simulink model "drone_propre"  (Simulink 6.1)
settings: Solver=ode45  StartTime=0.0  StopTime=10.0  RelTol=1e-3
undefined symbols (not defined in the file): Mecanique
libraries: mblibv1 x15, powerlib x2, electricdrivelib x1
settings Model: LastModifiedBy=Vincent
settings DebuggingCC: SolverPrmCheckMsg=warning

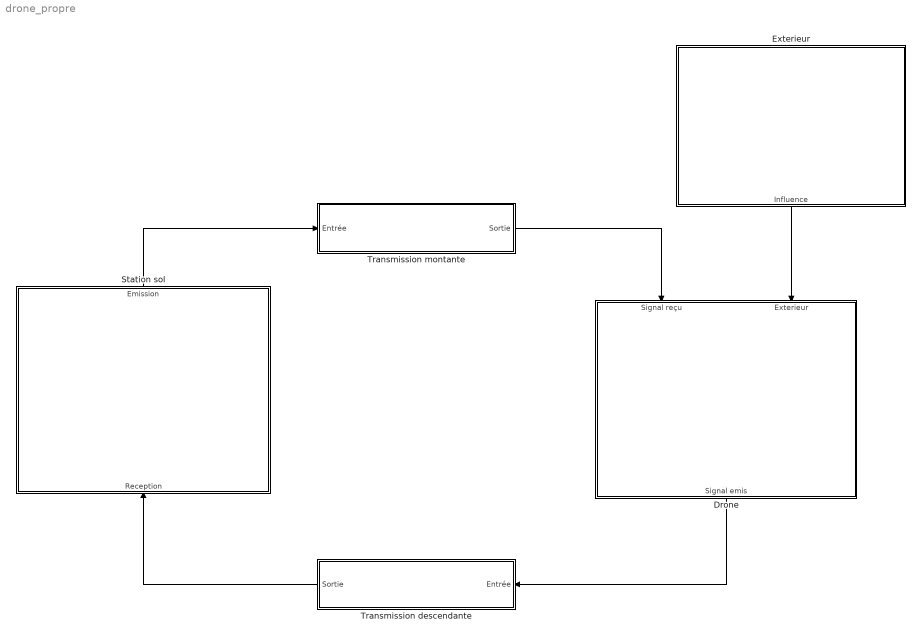
== system drone_propre ==
  Drone : Subsystem  Orientation=down
      mask Display: image(imread('C:\Projets\CMD\Simulations\Propre\images\drone.jpg'))
  Exterieur : Subsystem  Orientation=down
      mask Display: image(imread('C:\Projets\CMD\Simulations\Propre\images\ciel.jpg'))
  Station sol : Subsystem  Orientation=up
      mask Display: image(imread('C:\Projets\CMD\Simulations\Propre\images\stationsol.jpg'))
  Transmission descendante : Subsystem  Orientation=left
      mask Display: image(imread('C:\Projets\CMD\Simulations\Propre\images\ondes2.jpg'))
  Transmission montante : Subsystem
      mask Display: image(imread('C:\Projets\CMD\Simulations\Propre\images\ondes1.jpg'))
  wires:
  Transmission descendante/1(Sortie) -> Station sol/1(Reception)
  Station sol/1(Emission) -> Transmission montante/1(Entrée)
  Transmission montante/1(Sortie) -> Drone/1(Signal reçu)
  Drone/1(Signal emis) -> Transmission descendante/1(Entrée)
  Exterieur/1(Influence) -> Drone/2(Exterieur)

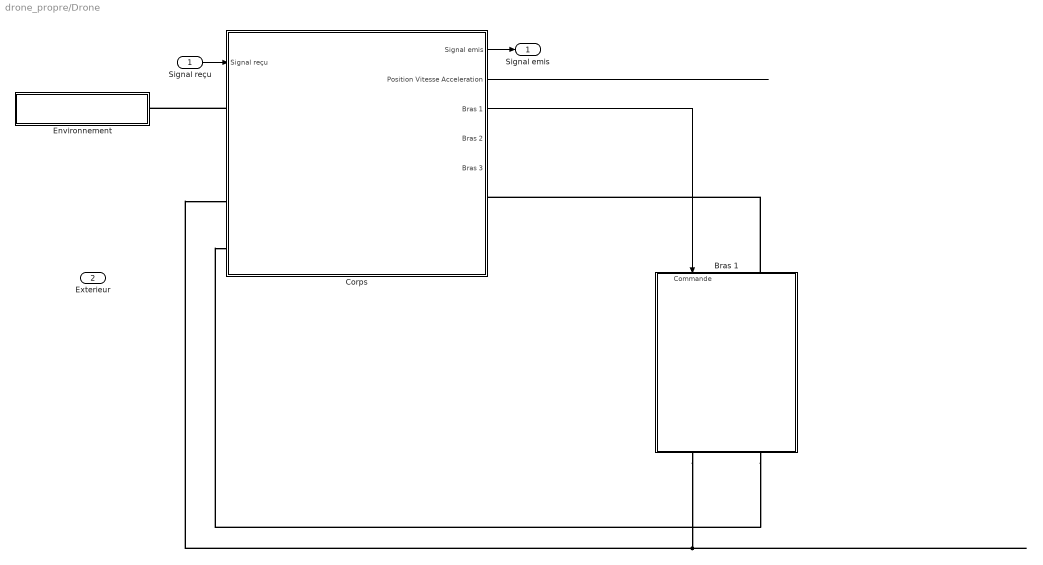
== system drone_propre/Drone ==
  Signal reçu : Inport  Port=1  LatchInput=off
  Exterieur : Inport  Port=2  LatchInput=off
  Bras 1 : Subsystem  Orientation=down
  Corps : Subsystem
  Environnement : Subsystem  Orientation=left
  Signal emis : Outport
  wires:
  Signal reçu/1 -> Corps/1(Signal reçu)
  Corps/1(Signal emis) -> Signal emis/1
  Corps/3(Bras 1) -> Bras 1/1(Commande)
  Corps/2(Position Vitesse Acceleration) -> ?
  connections:
  Corps/LConn1 -- Environnement/LConn1
  Corps/LConn3 -- Bras 1/RConn1
  Bras 1/RConn2 -- Corps/LConn4
  Bras 1/LConn1 -- Corps/RConn1

== system drone_propre/Exterieur ==
  Influence : Outport

== system drone_propre/Station sol ==
  Reception : Inport  Port=1  LatchInput=off
  Emission : Outport
  wires:
  Reception/1 -> Emission/1

== system drone_propre/Transmission descendante ==
  Entrée : Inport  Port=1  LatchInput=off
  Délai de transmission : TransportDelay  DelayTime=1E-4
  Sortie : Outport
  wires:
  Entrée/1 -> Délai de transmission/1
  Délai de transmission/1 -> Sortie/1

== system drone_propre/Transmission montante ==
  Entrée : Inport  Port=1  LatchInput=off
  Délai de transmission : TransportDelay  DelayTime=1E-4
  Sortie : Outport
  wires:
  Entrée/1 -> Délai de transmission/1
  Délai de transmission/1 -> Sortie/1

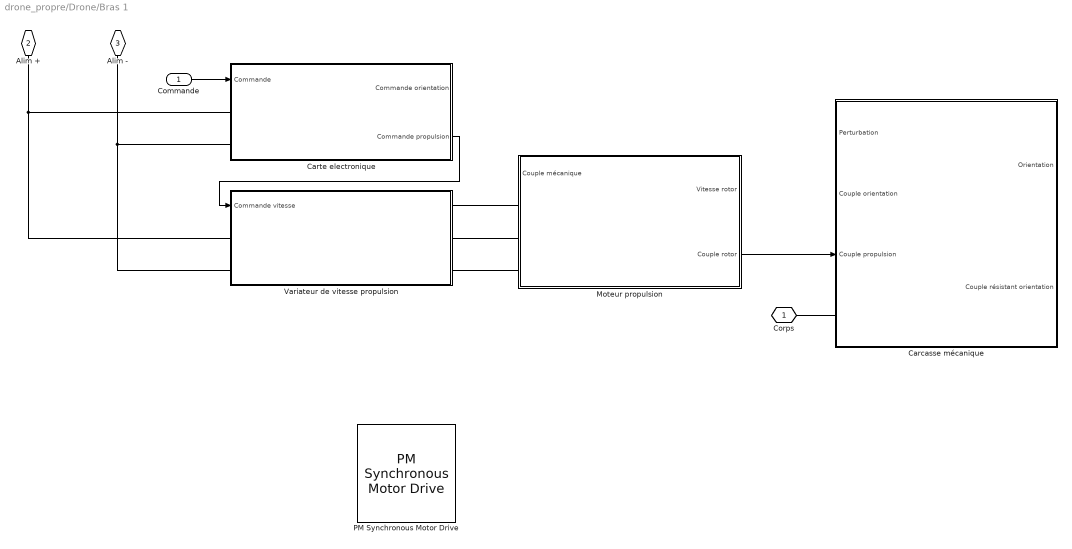
== system drone_propre/Drone/Bras 1 ==
  Commande : Inport  Port=1  LatchInput=off
  Carcasse mécanique : Subsystem
  Carte electronique : Subsystem
  Moteur propulsion : Subsystem
  PM Synchronous Motor Drive : electricdrivelib/AC drives/PM Synchronous Motor Drive
  Variateur de vitesse propulsion : Subsystem
  Corps : PMIOPort  Tag=PMCPort  Port=1  Side=Left
  Alim + : PMIOPort  Tag=PMCPort  Orientation=down  Port=2  Side=Right
  Alim - : PMIOPort  Tag=PMCPort  Orientation=down  Port=3  Side=Right
  wires:
  Moteur propulsion/2(Couple rotor) -> Carcasse mécanique/3(Couple propulsion)
  Commande/1 -> Carte electronique/1(Commande)
  Carte electronique/2(Commande propulsion) -> Variateur de vitesse propulsion/1(Commande vitesse)
  connections:
  Alim +/RConn1 -- Variateur de vitesse propulsion/LConn1 -- Carte electronique/LConn1
  Alim -/RConn1 -- Variateur de vitesse propulsion/LConn2 -- Carte electronique/LConn2
  Carcasse mécanique/LConn1 -- Corps/RConn1
  Moteur propulsion/LConn1 -- Variateur de vitesse propulsion/RConn1
  Variateur de vitesse propulsion/RConn2 -- Moteur propulsion/LConn2
  Moteur propulsion/LConn3 -- Variateur de vitesse propulsion/RConn3

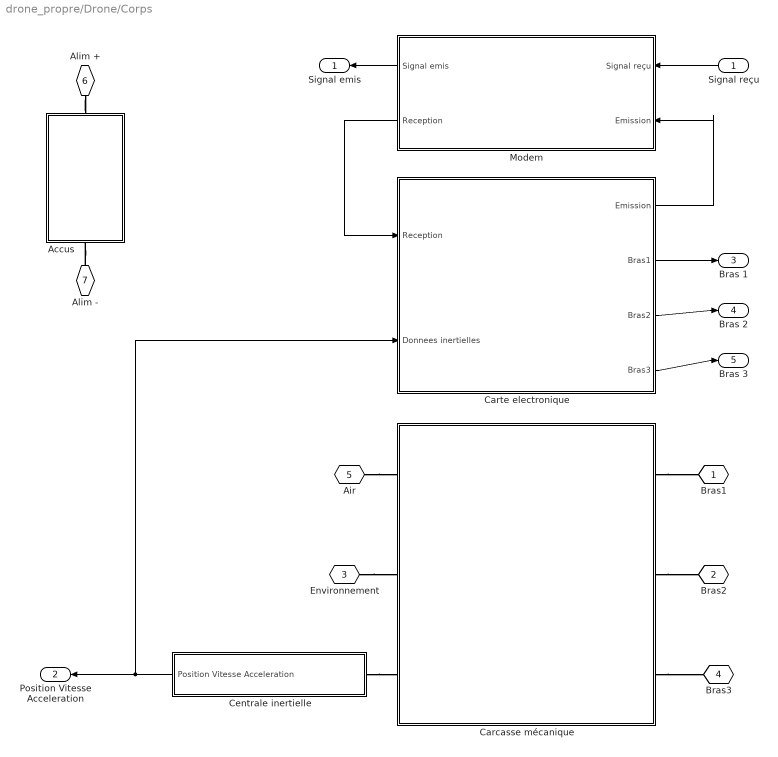
== system drone_propre/Drone/Corps ==
  Signal reçu : Inport  Orientation=left  Port=1  LatchInput=off
  Accus : Subsystem  Orientation=down
  Carcasse mécanique : Subsystem  Orientation=left
  Carte electronique : Subsystem
  Centrale inertielle : Subsystem  Orientation=left
  Modem : Subsystem  Orientation=left
  Bras1 : PMIOPort  Tag=PMCPort  Orientation=left  Port=1  Side=Right
  Bras2 : PMIOPort  Tag=PMCPort  Orientation=left  Port=2  Side=Right
  Environnement : PMIOPort  Tag=PMCPort  Port=3  Side=Left
  Bras3 : PMIOPort  Tag=PMCPort  Orientation=left  Port=4  Side=Right
  Air : PMIOPort  Tag=PMCPort  Port=5  Side=Left
  Alim + : PMIOPort  Tag=PMCPort  Orientation=down  Port=6  Side=Left
  Alim - : PMIOPort  Tag=PMCPort  Orientation=up  Port=7  Side=Left
  Signal emis : Outport  Orientation=left
  Position Vitesse Acceleration : Outport  Orientation=left  Port=2
  Bras 1 : Outport  Port=3
  Bras 2 : Outport  Port=4
  Bras 3 : Outport  Port=5
  wires:
  Centrale inertielle/1(Position Vitesse Acceleration) -> Position Vitesse Acceleration/1, Carte electronique/2(Donnees inertielles)
  Carte electronique/2(Bras1) -> Bras 1/1
  Carte electronique/3(Bras2) -> Bras 2/1
  Carte electronique/4(Bras3) -> Bras 3/1
  Modem/1(Signal emis) -> Signal emis/1
  Carte electronique/1(Emission) -> Modem/2("Emission ")
  Signal reçu/1 -> Modem/1(Signal reçu)
  Modem/2(Reception) -> Carte electronique/1(Reception)
  connections:
  Carcasse mécanique/LConn1 -- Bras1/RConn1
  Carcasse mécanique/LConn2 -- Bras2/RConn1
  Carcasse mécanique/LConn3 -- Bras3/RConn1
  Environnement/RConn1 -- Carcasse mécanique/RConn2
  Centrale inertielle/LConn1 -- Carcasse mécanique/RConn3
  Air/RConn1 -- Carcasse mécanique/RConn1
  Alim +/RConn1 -- Accus/LConn1
  Alim -/RConn1 -- Accus/RConn1

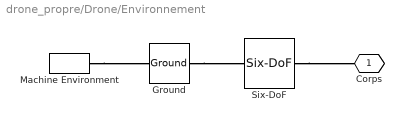
== system drone_propre/Drone/Environnement ==
  Ground : mblibv1/Bodies/Ground  Opaque=on  LeftPortType=env  RightPortType=workingframe  PhysicalDomain=Mechanical  DialogClass=GroundBlock  CoordPosition=[0 0 0]  CoordPositionUnits=m  StateVectorMgrId=-1  MachineId=[0 0]  ShowEnvPort=on
  Machine Environment : mblibv1/Bodies/Machine Environment  Tag=Factory ground  DialogController=MECH.DialogSource  Opaque=on  PortType=env  PhysicalDomain=Mechanical  DialogTemplateClass=MECH.MachineEnvironment  SyncWhenCopied=off  Gravity=Environnement.Gravite  GravityUnits=m/s^2  GravityAsSignal=off  Dimensionality=3D Only  AnalysisType=Forward dynamics  LinearAssemblyTolerance=1e-3  LinearAssemblyToleranceUnits=m  AngularAssemblyTolerance=1e-3  AngularAssemblyToleranceUnits=rad  ConstraintSolverType=Stabilizing  ConstraintRelTolerance=1e-4  ConstraintAbsTolerance=1e-4  UseRobustSingularityHandling=off  StatePerturbationType=Fixed  PerturbationSize=1e-5  VisualizeMachine=on
  Six-DoF : mblibv1/Joints/Six-DoF  PhysicalDomain=mechanical  SubClassName=Unknown  LeftPortType=blob  RightPortType=blob  LConnTagsString=__newl0  RConnTagsString=__newr0  NumSAPorts=0  CutJoint=off  MarkAsCut=off  Primitives=prismatic_prismatic_prismatic_spherical  PrimitiveProps=P1$INERTIAL$[1 0 0]$prismatic#P2$INERTIAL$[0 1 0]$prismatic#P3$INERTIAL$[0 0 1]$prismatic#S$INERTIAL$[0 0 0]$spherical  DialogClass=JointBlock
  Corps : PMIOPort  Tag=PMCPort  Orientation=left  Port=1  Side=Left
  connections:
  Ground/RConn1 -- Six-DoF/LConn1
  Machine Environment/RConn1 -- Ground/LConn1
  Six-DoF/RConn1 -- Corps/RConn1

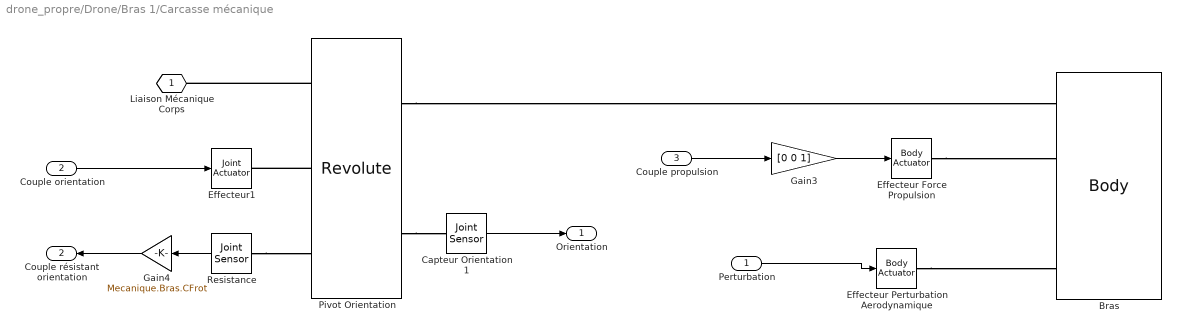
== system drone_propre/Drone/Bras 1/Carcasse mécanique ==
  Perturbation : Inport  Port=1  LatchInput=off
  Couple orientation : Inport  Port=2  LatchInput=off
  Couple propulsion : Inport  Port=3  LatchInput=off
  Bras : mblibv1/Bodies/Body  PhysicalDomain=mechanical  SubClassName=Unknown  LeftPortType=workingframe  RightPortType=workingframe  LConnTagsString=CS1|CS2|CS3|CS4  DialogClass=MechanicalBodyBlock  Mass=Mecanique.Bras.Masse  MassUnits=kg  InertiaUnits=kg*m^2  Inertia=Mecanique.Bras.Inertie  Shape=Cylinder  ShapeDims=[1 1]  ShapeUnits=m  ShapeUse=false  Density=1  DensityUnits=kg/m^3  DensityUse=false  CG=Left$CG$Mecanique.Longeur*[1 0 0]$CS1$CS1$m$[0 0 0]$Euler X-Y-Z$deg$CS1$false  WorkingFrames=Left$CS1$[0 0 0]$ADJOINING$ADJOINING$m$[0 0 0]$Euler X-Y-Z$deg$ADJOINING$true#Left$CS2$Mecanique.Longeur*[1 0 0]$CS1$CS1$m$[0 0 0]$Euler X-Y-Z$deg$CS1$true#Left$CS3$Mecanique.Longeur*[1 0 0]$CS1$CS1$m$[0 0 0]$Euler X-Y-Z$deg$CS1$true#Left$CS4$Mecanique.Longeur*[1 0 0]$CG$CG$m$[0 0 0]$Euler X-Y-Z$deg$WORLD$true
  Capteur Orientation 1 : mblibv1/Sensors &  Actuators/Joint Sensor  Opaque=on  PhysicalDomain=Mechanical  PortType=blob  Muxed=on  Pose=off  Angle=on  AngleUnits=rad  ArcVelocity=off  ArcVelocityUnits=rad/s  ArcAcceleration=off  ArcAccelerationUnits=rad/s^2  CoordPosition=on  CoordPositionUnits=m  Velocity=off  VelocityUnits=m/s  Acceleration=off  AccelerationUnits=m/s^2  Quaternion=on  QuaternionDT=off  QuaternionDDT=off  QuaternionUnits=off  OutputVector=[ 1 ]  ActiveIO=off  Width=1  DialogClass=MechanicalSensorBlock  Primitive=R1  Force=off  ForceUnits=N  Torque=off  TorqueUnits=N-m  ReferenceFrame=Absolute (INERTIAL)  ReactionSensedSide=Base  ReactionReferenceFrame=Local (Body CS)  ReactionForce=off  ReactionForceUnits=N  ReactionMoment=off  ReactionMomentUnits=N-m
  Effecteur Force Propulsion : mblibv1/Sensors &  Actuators/Body Actuator  Opaque=on  PhysicalDomain=Mechanical  PortType=blob  ActuationStyle=Force  AngleUnits=deg  ArcVelocityUnits=deg/s  ArcAccelerationUnits=deg/s^2  CoordPositionUnits=m  VelocityUnits=m/s  AccelerationUnits=m/s^2  ForceUnits=N  TorqueUnits=N-m  ActiveIO=off  Width=3  DialogClass=MechanicalActuatorBlock  ReferenceFrame=Local (Body CS)  Angle=off  CoordPosition=on  Force=on  Torque=off
  "Effecteur Perturbation Aerodynamique " : mblibv1/Sensors &  Actuators/Body Actuator  Opaque=on  PhysicalDomain=Mechanical  PortType=blob  ActuationStyle=Force  AngleUnits=deg  ArcVelocityUnits=deg/s  ArcAccelerationUnits=deg/s^2  CoordPositionUnits=m  VelocityUnits=m/s  AccelerationUnits=m/s^2  ForceUnits=N  TorqueUnits=N-m  ActiveIO=off  Width=6  DialogClass=MechanicalActuatorBlock  ReferenceFrame=Local (Body CS)  Angle=off  CoordPosition=on  Force=on  Torque=on
  Effecteur1 : mblibv1/Sensors &  Actuators/Joint Actuator  Opaque=on  PhysicalDomain=Mechanical  PortType=blob  ActuationStyle=Force  AngleUnits=deg  ArcVelocityUnits=deg/s  ArcAccelerationUnits=deg/s^2  CoordPositionUnits=m  VelocityUnits=m/s  AccelerationUnits=m/s^2  ForceUnits=N  TorqueUnits=N-m  ActiveIO=off  Width=1  DialogClass=MechanicalActuatorBlock  Primitive=R1  ReferenceFrame=Absolute (INERTIAL)
  Gain3 : Gain  Gain=[0 0 1]
  Gain4 : Gain  Orientation=left  Gain=Mecanique.Bras.CFrot  SaturateOnIntegerOverflow=on
  Pivot Orientation : mblibv1/Joints/Revolute  PhysicalDomain=mechanical  SubClassName=Unknown  LeftPortType=blob  RightPortType=blob  LConnTagsString=__newl0|SA1|SA2  RConnTagsString=__newr0|SA1  NumSAPorts=3  CutJoint=off  MarkAsCut=off  Primitives=revolute  PrimitiveProps=R1$Base$[1 0 0]$revolute  DialogClass=JointBlock
  Resistance : mblibv1/Sensors &  Actuators/Joint Sensor  Orientation=left  Opaque=on  PhysicalDomain=Mechanical  PortType=blob  Muxed=off  Pose=off  Angle=off  AngleUnits=rad  ArcVelocity=on  ArcVelocityUnits=rad/s  ArcAcceleration=off  ArcAccelerationUnits=rad/s^2  CoordPosition=on  CoordPositionUnits=m  Velocity=off  VelocityUnits=m/s  Acceleration=off  AccelerationUnits=m/s^2  Quaternion=on  QuaternionDT=off  QuaternionDDT=off  QuaternionUnits=off  OutputVector=[ 1 ]  ActiveIO=off  Width=1  DialogClass=MechanicalSensorBlock  Primitive=R1  Force=off  ForceUnits=N  Torque=off  TorqueUnits=N-m  ReferenceFrame=Absolute (INERTIAL)  ReactionSensedSide=Base  ReactionReferenceFrame=Local (Body CS)  ReactionForce=off  ReactionForceUnits=N  ReactionMoment=off  ReactionMomentUnits=N-m
  Liaison Mécanique Corps : PMIOPort  Tag=PMCPort  Port=1  Side=Left
  Orientation : Outport
  Couple résistant orientation : Outport  Orientation=left  Port=2
  wires:
  Resistance/1 -> Gain4/1
  Perturbation/1 -> "Effecteur Perturbation Aerodynamique "/1
  Capteur Orientation 1/1 -> Orientation/1
  Gain3/1 -> Effecteur Force Propulsion/1
  Couple orientation/1 -> Effecteur1/1
  Gain4/1 -> Couple résistant orientation/1
  Couple propulsion/1 -> Gain3/1
  connections:
  Resistance/LConn1 -- Pivot Orientation/LConn3
  Pivot Orientation/LConn2 -- Effecteur1/RConn1
  Pivot Orientation/LConn1 -- Liaison Mécanique Corps/RConn1
  Pivot Orientation/RConn1 -- Bras/LConn1
  Pivot Orientation/RConn2 -- Capteur Orientation 1/LConn1
  Effecteur Force Propulsion/RConn1 -- Bras/LConn2
  "Effecteur Perturbation Aerodynamique "/RConn1 -- Bras/LConn4

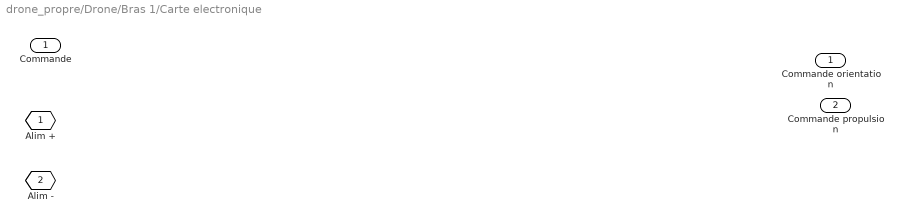
== system drone_propre/Drone/Bras 1/Carte electronique ==
  Commande : Inport  Port=1  LatchInput=off
  Alim + : PMIOPort  Tag=PMCPort  Port=1  Side=Left
  Alim - : PMIOPort  Tag=PMCPort  Port=2  Side=Left
  Commande orientation : Outport
  Commande propulsion : Outport  Port=2

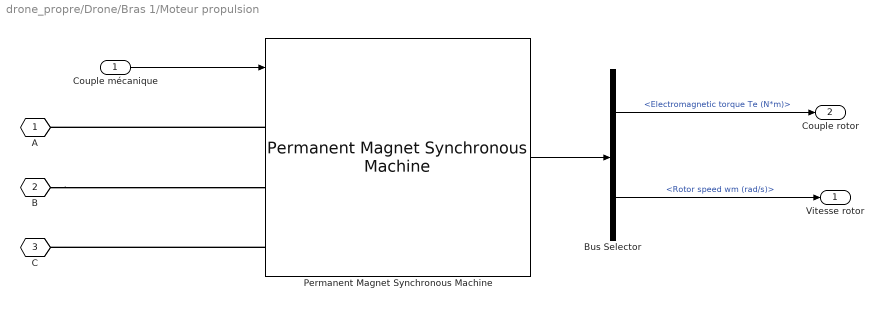
== system drone_propre/Drone/Bras 1/Moteur propulsion ==
  Couple mécanique : Inport  Port=1  LatchInput=off
  Bus Selector : BusSelector  DialogController=Simulink.DDGSource_Bus  OutputSignals=Electromagnetic torque Te (N*m),Rotor speed wm (rad/s)
  Permanent Magnet Synchronous Machine : powerlib/Machines/Permanent Magnet Synchronous Machine  PresetModel=No  ShowDetailedParameters=on  Resistance=2.8750  Inductances=[8.5e-3, 8.5e-3]  Flux=0.175  Mechanical="[ 0.8e-3, 0,  4 ]"
  A : PMIOPort  Tag=PMCPort  Port=1  Side=Left
  B : PMIOPort  Tag=PMCPort  Port=2  Side=Left
  C : PMIOPort  Tag=PMCPort  Port=3  Side=Left
  Vitesse rotor : Outport
  Couple rotor : Outport  Port=2
  wires:
  Permanent Magnet Synchronous Machine/1 -> Bus Selector/1
  Bus Selector/1 -> Couple rotor/1  "<Electromagnetic torque Te (N*m)>"
  Bus Selector/2 -> Vitesse rotor/1  "<Rotor speed wm (rad/s)>"
  Couple mécanique/1 -> Permanent Magnet Synchronous Machine/1
  connections:
  Permanent Magnet Synchronous Machine/LConn3 -- C/RConn1
  B/RConn1 -- Permanent Magnet Synchronous Machine/LConn2
  Permanent Magnet Synchronous Machine/LConn1 -- A/RConn1

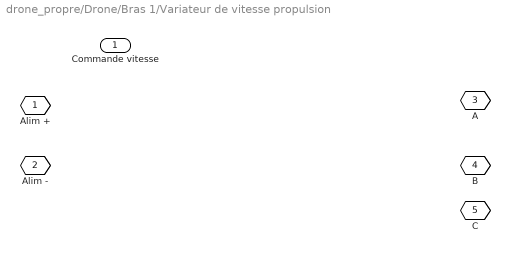
== system drone_propre/Drone/Bras 1/Variateur de vitesse propulsion ==
  Commande vitesse : Inport  Port=1  LatchInput=off
  Alim + : PMIOPort  Tag=PMCPort  Port=1  Side=Left
  Alim - : PMIOPort  Tag=PMCPort  Port=2  Side=Left
  A : PMIOPort  Tag=PMCPort  Orientation=left  Port=3  Side=Right
  B : PMIOPort  Tag=PMCPort  Orientation=left  Port=4  Side=Right
  C : PMIOPort  Tag=PMCPort  Orientation=left  Port=5  Side=Right

== system drone_propre/Drone/Corps/Accus ==
  DC Voltage Source : powerlib/Electrical Sources/DC Voltage Source  Orientation=up  Amplitude=15  Measurements=None
  Alim + : PMIOPort  Tag=PMCPort  Orientation=left  Port=1  Side=Left
  Alim - : PMIOPort  Tag=PMCPort  Orientation=left  Port=2  Side=Right
  connections:
  DC Voltage Source/RConn1 -- Alim +/RConn1
  Alim -/RConn1 -- DC Voltage Source/LConn1

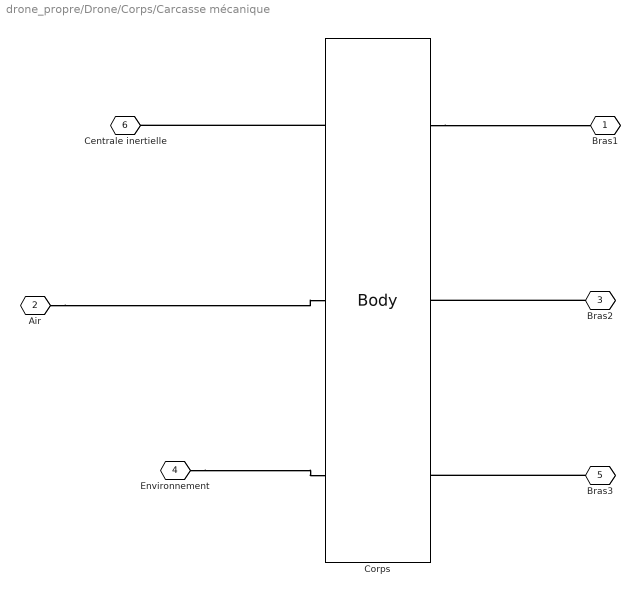
== system drone_propre/Drone/Corps/Carcasse mécanique ==
  Corps : mblibv1/Bodies/Body  PhysicalDomain=mechanical  SubClassName=Unknown  LeftPortType=workingframe  RightPortType=workingframe  LConnTagsString=CS4|CS7|CG  RConnTagsString=CS1|CS2|CS3  DialogClass=MechanicalBodyBlock  Mass=Mecanique.Corps.Masse  MassUnits=kg  InertiaUnits=kg*m^2  Inertia=Mecanique.Corps.Inertie  Shape=Cylinder  ShapeDims=[1 1]  ShapeUnits=m  ShapeUse=false  Density=1  DensityUnits=kg/m^3  DensityUse=false  CG=Left$CG$[0 0 0]$ADJOINING$ADJOINING$m$[0 0 0]$Euler X-Y-Z$deg$ADJOINING$true  WorkingFrames=Right$CS1$[0 0 0]$CG$CG$m$[0 0 0]$Euler Z-Y-X$deg$CG$true#Right$CS2$[0 0 0]$CG$CG$m$[120 0 0]$Euler Z-Y-X$deg$CG$true#Right$CS3$[0 0 0]$CG$CG$m$[240 0 0]$Euler Z-Y-X$deg$CG$true#Left$CS4$[0 0 0]$CG$CG$m$[0 0 0]$Euler X-Y-Z$deg$WORLD$true#Left$CS7$[0 0 0]$CG$CG$m$[0 0 0]$Euler X-Y-Z$deg$WORLD$true
  Bras1 : PMIOPort  Tag=PMCPort  Orientation=left  Port=1  Side=Left
  Air : PMIOPort  Tag=PMCPort  Port=2  Side=Right
  Bras2 : PMIOPort  Tag=PMCPort  Orientation=left  Port=3  Side=Left
  Environnement : PMIOPort  Tag=PMCPort  Port=4  Side=Right
  Bras3 : PMIOPort  Tag=PMCPort  Orientation=left  Port=5  Side=Left
  Centrale inertielle : PMIOPort  Tag=PMCPort  Port=6  Side=Right
  connections:
  Corps/RConn1 -- Bras1/RConn1
  Bras2/RConn1 -- Corps/RConn2
  Bras3/RConn1 -- Corps/RConn3
  Environnement/RConn1 -- Corps/LConn3
  Air/RConn1 -- Corps/LConn2
  Corps/LConn1 -- Centrale inertielle/RConn1

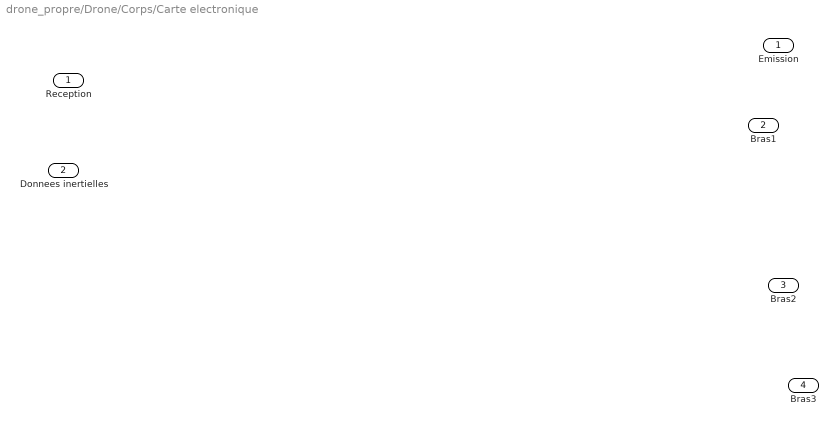
== system drone_propre/Drone/Corps/Carte electronique ==
  Reception : Inport  Port=1  LatchInput=off
  Donnees inertielles : Inport  Port=2  LatchInput=off
  Emission : Outport
  Bras1 : Outport  Port=2
  Bras2 : Outport  Port=3
  Bras3 : Outport  Port=4

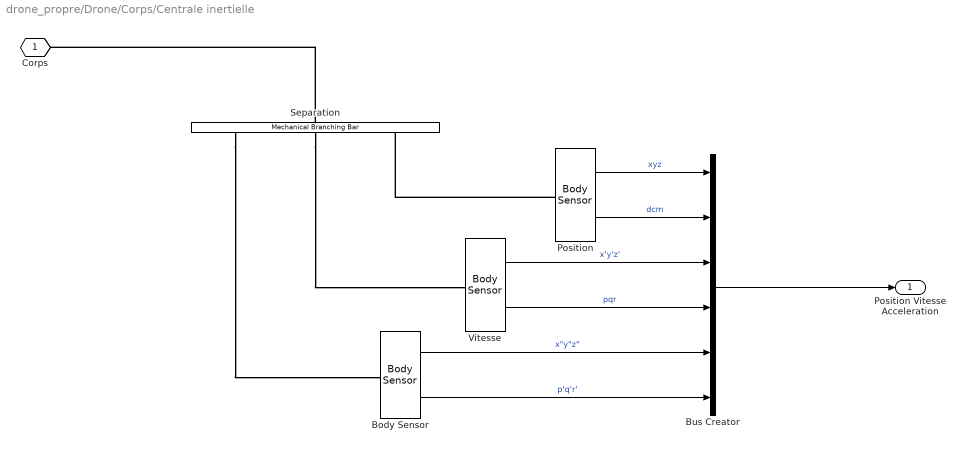
== system drone_propre/Drone/Corps/Centrale inertielle ==
  Body Sensor : mblibv1/Sensors &  Actuators/Body Sensor  Opaque=on  PhysicalDomain=Mechanical  PortType=blob  Muxed=off  Pose=off  Angle=on  AngleUnits=deg  ArcVelocity=off  ArcVelocityUnits=deg/s  ArcAcceleration=on  ArcAccelerationUnits=rad/s^2  CoordPosition=off  CoordPositionUnits=m  Velocity=off  VelocityUnits=m/s  Acceleration=on  AccelerationUnits=m/s^2  Quaternion=on  QuaternionDT=off  QuaternionDDT=off  QuaternionUnits=off  OutputVector=[ 3 3 ]  ActiveIO=off  Width=12  DialogClass=MechanicalSensorBlock  ReferenceFrame=Absolute (World)
  Bus Creator : BusCreator  DialogController=Simulink.DDGSource_Bus  Inputs=6
  Position : mblibv1/Sensors &  Actuators/Body Sensor  Opaque=on  PhysicalDomain=Mechanical  PortType=blob  Muxed=off  Pose=on  Angle=on  AngleUnits=deg  ArcVelocity=off  ArcVelocityUnits=deg/s  ArcAcceleration=off  ArcAccelerationUnits=deg/s^2  CoordPosition=on  CoordPositionUnits=m  Velocity=off  VelocityUnits=m/s  Acceleration=off  AccelerationUnits=m/s^2  Quaternion=on  QuaternionDT=off  QuaternionDDT=off  QuaternionUnits=off  OutputVector=[ 3 9 ]  ActiveIO=off  Width=12  DialogClass=MechanicalSensorBlock  ReferenceFrame=Absolute (World)
  Separation : mblibv1/Utilities/Mechanical Branching Bar  Orientation=down  PhysicalDomain=mechanical  SubClassName=Unknown  LeftPortType=blob  RightPortType=blob  LConnTagsString=_newl0  RConnTagsString=SA0|SA1|SA2  DialogClass=MechanicalBranchingBarBlock  NumSAPorts=3
  Vitesse : mblibv1/Sensors &  Actuators/Body Sensor  Opaque=on  PhysicalDomain=Mechanical  PortType=blob  Muxed=off  Pose=off  Angle=on  AngleUnits=deg  ArcVelocity=on  ArcVelocityUnits=rad/s  ArcAcceleration=off  ArcAccelerationUnits=deg/s^2  CoordPosition=off  CoordPositionUnits=m  Velocity=on  VelocityUnits=m/s  Acceleration=off  AccelerationUnits=m/s^2  Quaternion=on  QuaternionDT=off  QuaternionDDT=off  QuaternionUnits=off  OutputVector=[ 3 3 ]  ActiveIO=off  Width=12  DialogClass=MechanicalSensorBlock  ReferenceFrame=Absolute (World)
  Corps : PMIOPort  Tag=PMCPort  Port=1  Side=Left
  Position Vitesse Acceleration : Outport
  wires:
  Position/1 -> Bus Creator/1  "xyz"
  Bus Creator/1 -> Position Vitesse Acceleration/1
  Position/2 -> Bus Creator/2  "dcm"
  Vitesse/1 -> Bus Creator/3  "x'y'z'"
  Vitesse/2 -> Bus Creator/4  "pqr"
  Body Sensor/1 -> Bus Creator/5  "x\"y\"z\""
  Body Sensor/2 -> Bus Creator/6  "p'q'r'"
  connections:
  Separation/LConn1 -- Corps/RConn1
  Position/LConn1 -- Separation/RConn3
  Separation/RConn2 -- Vitesse/LConn1
  Separation/RConn1 -- Body Sensor/LConn1

== system drone_propre/Drone/Corps/Modem ==
  Signal reçu : Inport  Port=1  LatchInput=off
  "Emission " : Inport  Port=2  LatchInput=off
  Signal emis : Outport
  Reception : Outport  Port=2
  wires:
  "Emission "/1 -> Signal emis/1
  Signal reçu/1 -> Reception/1
